simulink model "simulink_robo_fixo"  (R2014a)
settings: Solver=ode45  StartTime=0.0  StopTime=Tsim  RelTol=1e-3
values from neighbouring files (symbols this model uses):
  a = 0.0    (= 0)    [simula_robo_fixo.m]
  b = 0.2    [simula_robo_fixo.m]
  Ic = 1    [simula_robo_fixo.m]
  Kp = u(1)    [sfunc_adaptativo_J.m]    (also in simula_robo_fixo.m = 0.05)
  m = 10    [simula_robo_fixo.m]
  r = 0.07    [simula_robo_fixo.m]
  thetao = 0.0    (= 0)    [simula_robo_fixo.m]
  Ts = 0.1    [simula_robo_fixo.m]
  xo = -1.5    [simula_robo_fixo.m]
  yo = -2.5    [simula_robo_fixo.m]
libraries: vrlib x1
settings Model: PauseTimes=9  Creator=Fabricio  LastModifiedBy=Thiago Lobo
settings DataIOCC: SignalLoggingSaveFormat=ModelDataLogs
settings DebuggingCC: UnderspecifiedInitializationDetection=Classic  MultiTaskDSMMsg=warning  MultiTaskCondExecSysMsg=none  StateNameClashWarn=warning
settings RTWCC: IncludeERTFirstTime=on

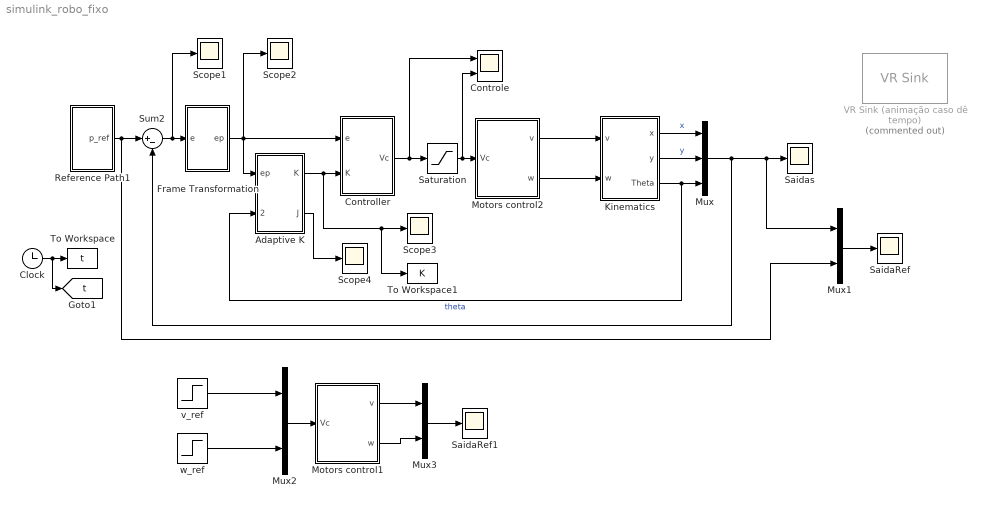
== system simulink_robo_fixo ==
  Adaptive K : Subsystem
  Clock : Clock
  Controle : Scope  NumInputPorts=2
      settings: ShowLegends=on  TimeRange=10  YMin=-5~-1e-08  YMax=20~1.3e-08  SaveName=ScopeData11
  Controller : Subsystem
  Frame Transformation : Subsystem
  Kinematics : Subsystem
  Motors control1 : Subsystem
  Motors control2 : Subsystem
  Mux : Mux  Inputs=3
  Mux1 : Mux  Inputs=2
  Mux2 : Mux  Inputs=2
  Mux3 : Mux  Inputs=2
  Reference Path1 : Subsystem
  SaidaRef : Scope
      settings: ShowLegends=on  TimeRange=10  YMin=-7.5  YMax=27.5  SaveName=ScopeData16
  SaidaRef1 : Scope
      settings: ShowLegends=on  TimeRange=10  YMin=-7.5  YMax=27.5  SaveName=ScopeData6
  Saidas : Scope
      settings: ShowLegends=on  TimeRange=10  YMax=100
  Saturation : Saturate  UpperLimit=[inf inf]  LowerLimit=-[inf inf]
  Scope{1..4} (4 alike) : Scope
      Scope1 settings: ShowLegends=on  TimeRange=10  SaveName=ScopeData2
      Scope2 settings: ShowLegends=on  TimeRange=10  SaveName=ScopeData9
      Scope3 settings: ShowLegends=on  TimeRange=10  YMax=300  SaveName=ScopeData4
      Scope4 settings: ShowLegends=on  TimeRange=10  SaveName=ScopeData8
  Sum2 : Sum  Inputs=|+-  SampleTime=Ts
  To Workspace : ToWorkspace  VariableName=t  SampleTime=Ts
  To Workspace1 : ToWorkspace  VariableName=K  SampleTime=Ts
  VR Sink (animação caso dê tempo) : vrlib/VR Sink  Commented=on  InstantiateOnLoad=on  SampleTime=0.1  ViewEnable=on  RemoteChange=off  RemoteView=on  AutoView=off  VideoDimensions=[]  AllowVariableSize=off
  v_ref : Step  Time=10  SampleTime=Ts
  w_ref : Step  Time=20  After=pi/2  SampleTime=Ts
  tag scope: t=global
  wires:
  Kinematics/2(y) -> Mux/2  "y"
  Kinematics/3(Theta) -> Adaptive K/2(Theta), Mux/3  "theta"
  Controller/1(Vc) -> Controle/1, Saturation/1
  Clock/1 -> To Workspace/1, [t]
  Mux/1 -> Mux1/1, Saidas/1, Sum2/2
  Sum2/1 -> Frame Transformation/1(e), Scope1/1
  Kinematics/1(x) -> Mux/1  "x"
  Motors control2/2(w) -> Kinematics/2(w)
  Motors control2/1(v) -> Kinematics/1(v)
  Frame Transformation/1(ep) -> Scope2/1, Adaptive K/1(ep), Controller/1(e)
  Adaptive K/2(J) -> Scope4/1
  Saturation/1 -> Motors control2/1(Vc), Controle/2
  Reference Path1/1(p_ref) -> Mux1/2, Sum2/1
  Mux1/1 -> SaidaRef/1
  Mux2/1 -> Motors control1/1(Vc)
  v_ref/1 -> Mux2/1
  w_ref/1 -> Mux2/2
  Mux3/1 -> SaidaRef1/1
  Motors control1/1(v) -> Mux3/1
  Motors control1/2(w) -> Mux3/2
  Adaptive K/1(K) -> To Workspace1/1, Scope3/1, Controller/2(K)

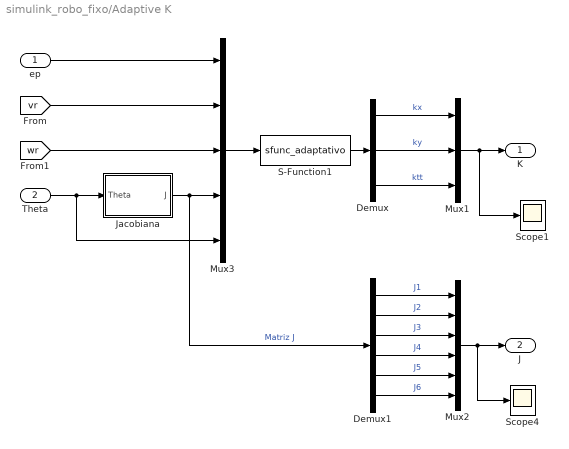
== system simulink_robo_fixo/Adaptive K ==
  ep : Inport
  Theta : Inport  Port=2
  Demux : Demux  Outputs=3
  Demux1 : Demux  Outputs=6
  Jacobiana : Subsystem
  Mux1 : Mux  Inputs=3
  Mux2 : Mux  Inputs=6
  Mux3 : Mux  Inputs=5
  S-Function1 : S-Function  FunctionName=sfunc_adaptativo  Parameters=Ts  EnableBusSupport=off
  Scope1 : Scope
      settings: ShowLegends=on  TimeRange=10  YMin=-100  YMax=220  SaveName=ScopeData14
  Scope4 : Scope
      settings: ShowLegends=on  TimeRange=10  SaveName=ScopeData13
  K : Outport
  J : Outport  Port=2
  wires:
  Mux3/1 -> S-Function1/1
  [vr] -> Mux3/2
  [wr] -> Mux3/3
  S-Function1/1 -> Demux/1
  Demux/3 -> Mux1/3  "ktt"
  Demux/2 -> Mux1/2  "ky"
  Demux/1 -> Mux1/1  "kx"
  ep/1 -> Mux3/1
  Theta/1 -> Mux3/5, Jacobiana/1(Theta)
  Jacobiana/1(J) -> Demux1/1, Mux3/4  "Matriz J"
  Demux1/3 -> Mux2/3  "J3"
  Demux1/2 -> Mux2/2  "J2"
  Demux1/1 -> Mux2/1  "J1"
  Demux1/4 -> Mux2/4  "J4"
  Demux1/5 -> Mux2/5  "J5"
  Demux1/6 -> Mux2/6  "J6"
  Mux1/1 -> Scope1/1, K/1
  Mux2/1 -> Scope4/1, J/1

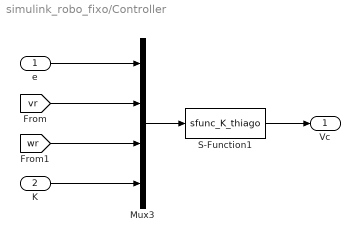
== system simulink_robo_fixo/Controller ==
  e : Inport
  K : Inport  Port=2
  Mux3 : Mux
  S-Function1 : S-Function  FunctionName=sfunc_K_thiago  Parameters=Ts  EnableBusSupport=off
  Vc : Outport
  wires:
  Mux3/1 -> S-Function1/1
  [vr] -> Mux3/2
  [wr] -> Mux3/3
  S-Function1/1 -> Vc/1
  e/1 -> Mux3/1
  K/1 -> Mux3/4

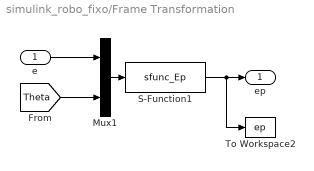
== system simulink_robo_fixo/Frame Transformation ==
  e : Inport
  Mux1 : Mux  Inputs=2
  S-Function1 : S-Function  FunctionName=sfunc_Ep  Parameters=Ts  EnableBusSupport=off
  To Workspace2 : ToWorkspace  VariableName=ep  SampleTime=Ts
  ep : Outport
  wires:
  S-Function1/1 -> To Workspace2/1, ep/1
  Mux1/1 -> S-Function1/1
  e/1 -> Mux1/1
  [Theta] -> Mux1/2

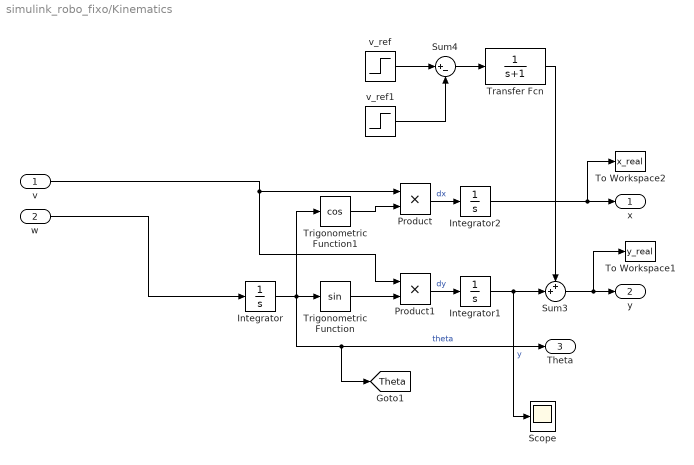
== system simulink_robo_fixo/Kinematics ==
  v : Inport
  w : Inport  Port=2
  Integrator : Integrator  InitialCondition=thetao
  Integrator1 : Integrator  InitialCondition=yo
  Integrator2 : Integrator  InitialCondition=xo
  Product : Product
  Product1 : Product
  Scope : Scope
      settings: TimeRange=10
  Sum3 : Sum  Inputs=++|
  Sum4 : Sum  Inputs=|+-
  To Workspace1 : ToWorkspace  VariableName=y_real  SampleTime=Ts
  To Workspace2 : ToWorkspace  VariableName=x_real  SampleTime=Ts
  Transfer Fcn : TransferFcn  Denominator=[1 1]
  Trigonometric Function : Trigonometry
  Trigonometric Function1 : Trigonometry  Operator=cos
  v_ref : Step  Time=80000  After=-0.1  SampleTime=Ts
  v_ref1 : Step  Time=810000  After=-0.1  SampleTime=Ts
  x : Outport
  y : Outport  Port=2
  Theta : Outport  Port=3
  tag scope: Theta=global
  wires:
  Trigonometric Function1/1 -> Product/2
  Product/1 -> Integrator2/1  "dx"
  Integrator/1 -> [Theta], Theta/1, Trigonometric Function1/1, Trigonometric Function/1  "theta"
  Integrator1/1 -> Sum3/2, Scope/1  "y"
  Product1/1 -> Integrator1/1  "dy"
  Trigonometric Function/1 -> Product1/2
  v_ref/1 -> Sum4/1
  v_ref1/1 -> Sum4/2
  Sum4/1 -> Transfer Fcn/1
  Integrator2/1 -> To Workspace2/1, x/1
  Sum3/1 -> To Workspace1/1, y/1
  Transfer Fcn/1 -> Sum3/1
  w/1 -> Integrator/1
  v/1 -> Product1/1, Product/1

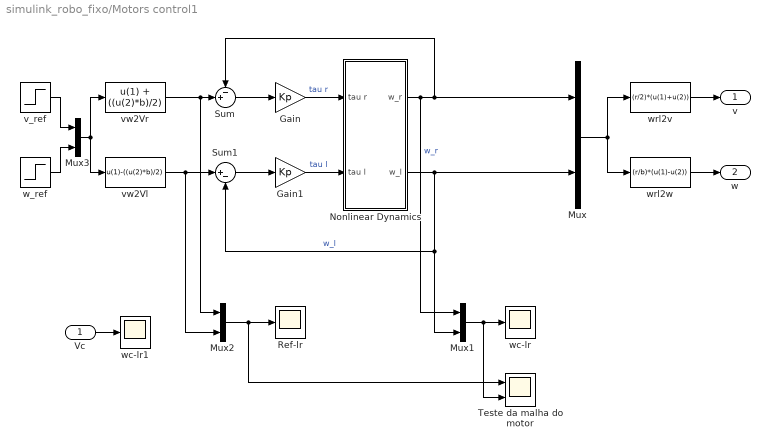
== system simulink_robo_fixo/Motors control1 ==
  Vc : Inport
  Gain : Gain  Gain=Kp
  Gain1 : Gain  Gain=Kp
  Mux{,1..3} (4 alike) : Mux  Inputs=2
  Nonlinear Dynamics : Subsystem
  Ref-lr : Scope
      settings: YMax=20  SaveName=ScopeData7
  Sum : Sum  Inputs=-+|
  Sum1 : Sum  Inputs=|+-
  Teste da malha do motor : Scope  NumInputPorts=2
      settings: YMin=-5~-5  YMax=5~5  SaveName=ScopeData10
  v_ref : Step  Time=10  SampleTime=Ts
  vw2Vl : Fcn  Expr=u(1)-((u(2)*b)/2)
  vw2Vr : Fcn  Expr=u(1) + ((u(2)*b)/2)
  w_ref : Step  Time=12  After=pi/2  SampleTime=Ts
  wc-lr : Scope
      settings: YMax=20  SaveName=ScopeData5
  wc-lr1 : Scope
      settings: YMax=20  SaveName=ScopeData3
  wrl2v : Fcn  Expr=(r/2)*(u(1)+u(2))
  wrl2w : Fcn  Expr=(r/b)*(u(1)-u(2))
  v : Outport
  w : Outport  Port=2
  wires:
  Gain/1 -> Nonlinear Dynamics/1(tau r)  "tau r"
  Sum/1 -> Gain/1
  Gain1/1 -> Nonlinear Dynamics/2(tau l)  "tau l"
  Sum1/1 -> Gain1/1
  Nonlinear Dynamics/1(w_r) -> Mux/1, Sum/1, Mux1/1  "w_r"
  Nonlinear Dynamics/2(w_l) -> Mux1/2, Sum1/2, Mux/2  "w_l"
  vw2Vr/1 -> Mux2/1, Sum/2
  vw2Vl/1 -> Sum1/1, Mux2/2
  Mux1/1 -> Teste da malha do motor/2, wc-lr/1
  Mux2/1 -> Teste da malha do motor/1, Ref-lr/1
  Mux/1 -> wrl2w/1, wrl2v/1
  wrl2v/1 -> v/1
  wrl2w/1 -> w/1
  w_ref/1 -> Mux3/2
  v_ref/1 -> Mux3/1
  Mux3/1 -> vw2Vl/1, vw2Vr/1
  Vc/1 -> wc-lr1/1

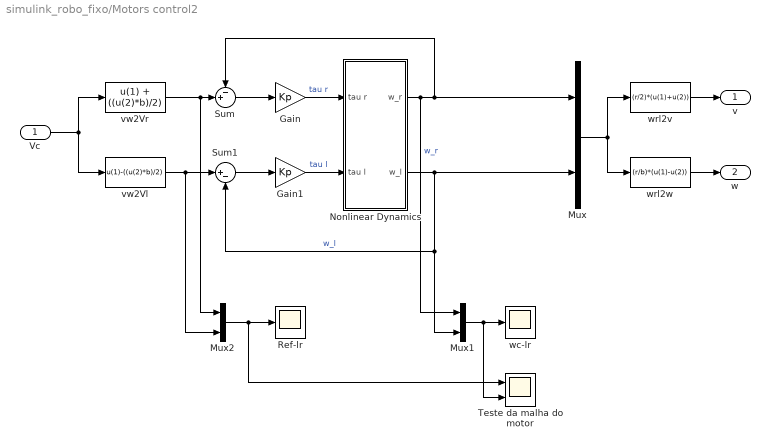
== system simulink_robo_fixo/Motors control2 ==
  Vc : Inport
  Gain : Gain  Gain=Kp
  Gain1 : Gain  Gain=Kp
  Mux : Mux  Inputs=2
  Mux1 : Mux  Inputs=2
  Mux2 : Mux  Inputs=2
  Nonlinear Dynamics : Subsystem
  Ref-lr : Scope
      settings: YMax=20  SaveName=ScopeData7
  Sum : Sum  Inputs=-+|
  Sum1 : Sum  Inputs=|+-
  Teste da malha do motor : Scope  NumInputPorts=2
      settings: YMin=-5~-5  YMax=5~5  SaveName=ScopeData10
  vw2Vl : Fcn  Expr=u(1)-((u(2)*b)/2)
  vw2Vr : Fcn  Expr=u(1) + ((u(2)*b)/2)
  wc-lr : Scope
      settings: YMax=20  SaveName=ScopeData5
  wrl2v : Fcn  Expr=(r/2)*(u(1)+u(2))
  wrl2w : Fcn  Expr=(r/b)*(u(1)-u(2))
  v : Outport
  w : Outport  Port=2
  wires:
  Gain/1 -> Nonlinear Dynamics/1(tau r)  "tau r"
  Sum/1 -> Gain/1
  Gain1/1 -> Nonlinear Dynamics/2(tau l)  "tau l"
  Sum1/1 -> Gain1/1
  Nonlinear Dynamics/1(w_r) -> Mux/1, Sum/1, Mux1/1  "w_r"
  Nonlinear Dynamics/2(w_l) -> Mux1/2, Sum1/2, Mux/2  "w_l"
  vw2Vr/1 -> Mux2/1, Sum/2
  vw2Vl/1 -> Sum1/1, Mux2/2
  Mux1/1 -> Teste da malha do motor/2, wc-lr/1
  Mux2/1 -> Teste da malha do motor/1, Ref-lr/1
  Mux/1 -> wrl2w/1, wrl2v/1
  wrl2v/1 -> v/1
  wrl2w/1 -> w/1
  Vc/1 -> vw2Vr/1, vw2Vl/1

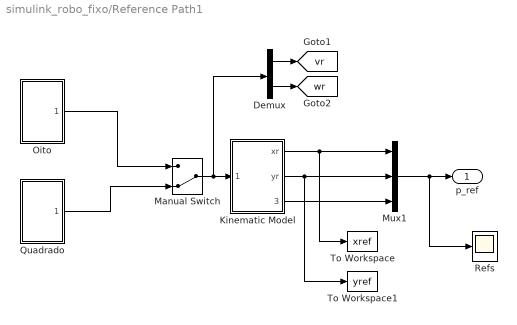
== system simulink_robo_fixo/Reference Path1 ==
  Demux : Demux  Outputs=2
  Kinematic Model : Subsystem
  Manual Switch : ManualSwitch  CurrentSetting=0
  Mux1 : Mux  Inputs=3
  Oito : Subsystem
  Quadrado : Subsystem
  Refs : Scope
      settings: ShowLegends=on  TimeRange=10  SaveName=ScopeData12
  To Workspace : ToWorkspace  VariableName=xref  SampleTime=Ts
  To Workspace1 : ToWorkspace  VariableName=yref  SampleTime=Ts
  p_ref : Outport
  tag scope: vr=global, wr=global
  wires:
  Kinematic Model/1(xr) -> To Workspace/1, Mux1/1
  Kinematic Model/3(thetar) -> Mux1/3
  Mux1/1 -> Refs/1, p_ref/1
  Kinematic Model/2(yr) -> To Workspace1/1, Mux1/2
  Oito/1(vw_ref) -> Manual Switch/1
  Quadrado/1(vw_ref) -> Manual Switch/2
  Demux/1 -> [vr]
  Demux/2 -> [wr]
  Manual Switch/1 -> Demux/1, Kinematic Model/1(vw_ref)

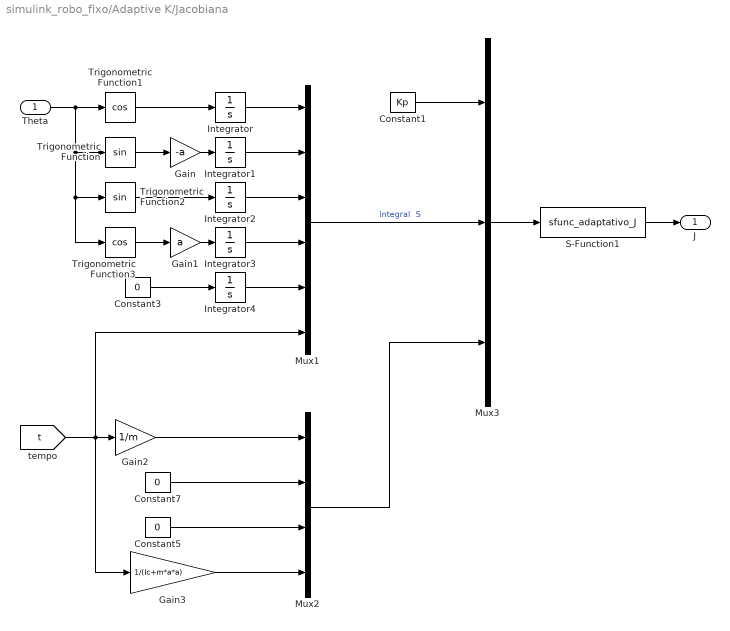
== system simulink_robo_fixo/Adaptive K/Jacobiana ==
  Theta : Inport
  Constant1 : Constant  Value=Kp  SampleTime=Ts
  Constant3 : Constant  Value=0  SampleTime=Ts
  Constant5 : Constant  Value=0  SampleTime=Ts
  Constant7 : Constant  Value=0  SampleTime=Ts
  Gain : Gain  Gain=-a
  Gain1 : Gain  Gain=a
  Gain2 : Gain  Gain=1/m
  Gain3 : Gain  Gain=1/(Ic+m*a*a)
  Integrator{,1..4} (5 alike) : Integrator
  Mux1 : Mux  Inputs=6
  Mux2 : Mux
  Mux3 : Mux  Inputs=3
  S-Function1 : S-Function  FunctionName=sfunc_adaptativo_J  Parameters=Ts  EnableBusSupport=off
  Trigonometric Function : Trigonometry
  Trigonometric Function1 : Trigonometry  Operator=cos
  Trigonometric Function2 : Trigonometry
  Trigonometric Function3 : Trigonometry  Operator=cos
  J : Outport
  wires:
  Mux3/1 -> S-Function1/1
  S-Function1/1 -> J/1
  Constant3/1 -> Integrator4/1
  Trigonometric Function1/1 -> Integrator/1
  Integrator/1 -> Mux1/1
  Integrator2/1 -> Mux1/3
  Integrator3/1 -> Mux1/4
  Integrator4/1 -> Mux1/5
  Integrator1/1 -> Mux1/2
  Gain2/1 -> Mux2/1
  Constant5/1 -> Mux2/3
  Gain3/1 -> Mux2/4
  Constant7/1 -> Mux2/2
  [t] -> Gain2/1, Mux1/6, Gain3/1
  Trigonometric Function/1 -> Gain/1
  Gain/1 -> Integrator1/1
  Theta/1 -> Trigonometric Function1/1, Trigonometric Function/1, Trigonometric Function2/1, Trigonometric Function3/1
  Trigonometric Function2/1 -> Integrator2/1
  Trigonometric Function3/1 -> Gain1/1
  Gain1/1 -> Integrator3/1
  Constant1/1 -> Mux3/1
  Mux1/1 -> Mux3/2  "integral  S"
  Mux2/1 -> Mux3/3

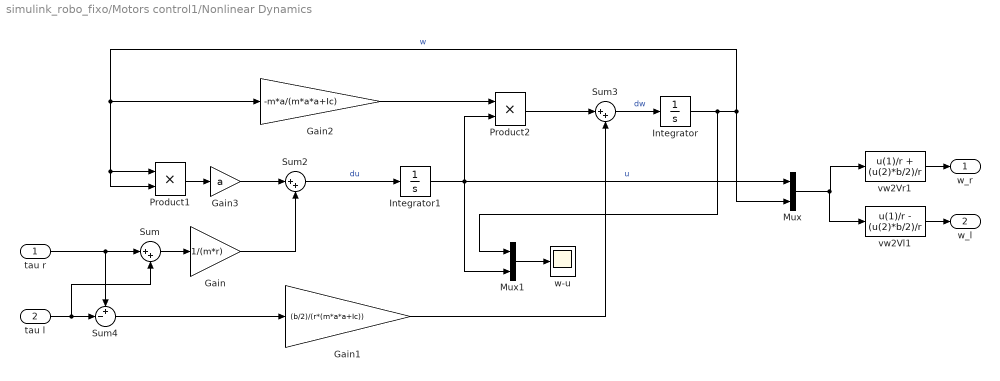
== system simulink_robo_fixo/Motors control1/Nonlinear Dynamics ==
  tau r : Inport
  tau l : Inport  Port=2
  Gain : Gain  Gain=1/(m*r)
  Gain1 : Gain  Gain=(b/2)/(r*(m*a*a+Ic))
  Gain2 : Gain  Gain=-m*a/(m*a*a+Ic)
  Gain3 : Gain  Gain=a
  Integrator : Integrator
  Integrator1 : Integrator
  Mux : Mux  Inputs=2
  Mux1 : Mux  Inputs=2
  Product1 : Product
  Product2 : Product  SampleTime=Ts
  Sum : Sum  Inputs=|++
  Sum2 : Sum  Inputs=|++
  Sum3 : Sum  Inputs=|++
  Sum4 : Sum  Inputs=+-|
  vw2Vl1 : Fcn  Expr=u(1)/r - (u(2)*b/2)/r
  vw2Vr1 : Fcn  Expr=u(1)/r + (u(2)*b/2)/r
  w-u : Scope
      settings: TimeRange=10  SaveName=ScopeData15
  w_r : Outport
  w_l : Outport  Port=2
  wires:
  tau r/1 -> Sum4/1, Sum/1
  Sum/1 -> Gain/1
  Product1/1 -> Gain3/1
  Gain3/1 -> Sum2/1
  Gain/1 -> Sum2/2
  Product2/1 -> Sum3/1
  Gain1/1 -> Sum3/2
  Integrator1/1 -> Mux1/2, Mux/1, Product2/2  "u"
  Sum2/1 -> Integrator1/1  "du"
  Sum3/1 -> Integrator/1  "dw"
  Integrator/1 -> Mux1/1, Mux/2, Gain2/1, Product1/1, Product1/2  "w"
  Gain2/1 -> Product2/1
  Sum4/1 -> Gain1/1
  tau l/1 -> Sum/2, Sum4/2
  vw2Vr1/1 -> w_r/1
  vw2Vl1/1 -> w_l/1
  Mux/1 -> vw2Vl1/1, vw2Vr1/1
  Mux1/1 -> w-u/1

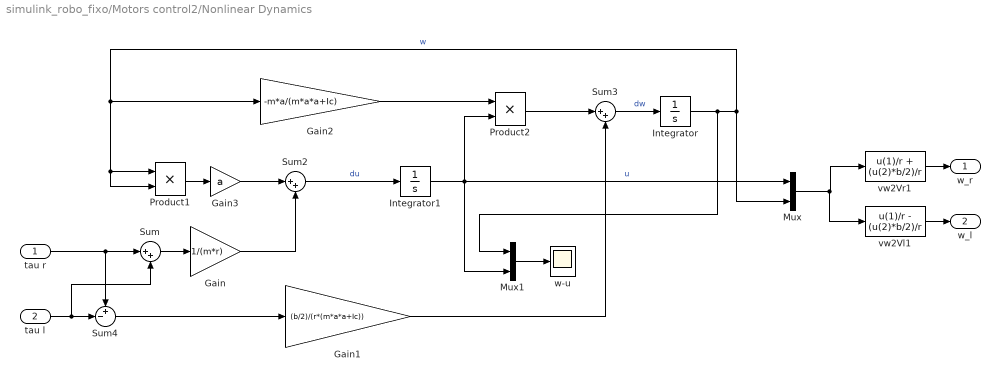
== system simulink_robo_fixo/Motors control2/Nonlinear Dynamics ==
  tau r : Inport
  tau l : Inport  Port=2
  Gain : Gain  Gain=1/(m*r)
  Gain1 : Gain  Gain=(b/2)/(r*(m*a*a+Ic))
  Gain2 : Gain  Gain=-m*a/(m*a*a+Ic)
  Gain3 : Gain  Gain=a
  Integrator : Integrator
  Integrator1 : Integrator
  Mux : Mux  Inputs=2
  Mux1 : Mux  Inputs=2
  Product1 : Product
  Product2 : Product  SampleTime=Ts
  Sum : Sum  Inputs=|++
  Sum2 : Sum  Inputs=|++
  Sum3 : Sum  Inputs=|++
  Sum4 : Sum  Inputs=+-|
  vw2Vl1 : Fcn  Expr=u(1)/r - (u(2)*b/2)/r
  vw2Vr1 : Fcn  Expr=u(1)/r + (u(2)*b/2)/r
  w-u : Scope
      settings: TimeRange=10  SaveName=ScopeData15
  w_r : Outport
  w_l : Outport  Port=2
  wires:
  tau r/1 -> Sum4/1, Sum/1
  Sum/1 -> Gain/1
  Product1/1 -> Gain3/1
  Gain3/1 -> Sum2/1
  Gain/1 -> Sum2/2
  Product2/1 -> Sum3/1
  Gain1/1 -> Sum3/2
  Integrator1/1 -> Mux1/2, Mux/1, Product2/2  "u"
  Sum2/1 -> Integrator1/1  "du"
  Sum3/1 -> Integrator/1  "dw"
  Integrator/1 -> Mux1/1, Mux/2, Gain2/1, Product1/1, Product1/2  "w"
  Gain2/1 -> Product2/1
  Sum4/1 -> Gain1/1
  tau l/1 -> Sum/2, Sum4/2
  vw2Vr1/1 -> w_r/1
  vw2Vl1/1 -> w_l/1
  Mux/1 -> vw2Vl1/1, vw2Vr1/1
  Mux1/1 -> w-u/1

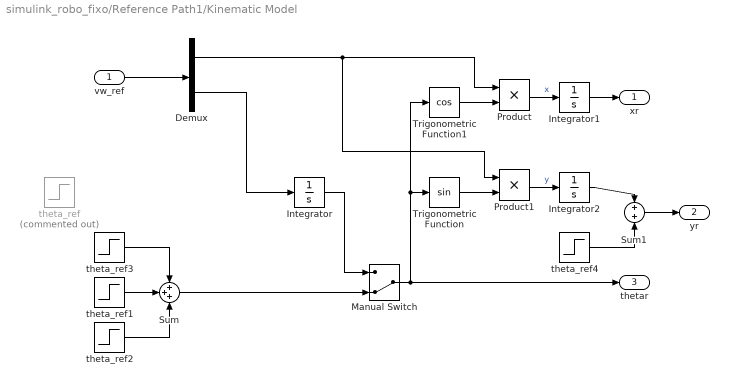
== system simulink_robo_fixo/Reference Path1/Kinematic Model ==
  vw_ref : Inport
  Demux : Demux  Outputs=2
  Integrator : Integrator
  Integrator1 : Integrator
  Integrator2 : Integrator
  Manual Switch : ManualSwitch  CurrentSetting=0
  Product : Product
  Product1 : Product
  Sum : Sum  Inputs=+++
  Sum1 : Sum
  Trigonometric Function : Trigonometry
  Trigonometric Function1 : Trigonometry  Operator=cos
  theta_ref : Step  Commented=on  Time=200  Before=pi/2  After=pi
  theta_ref1 : Step  Time=20  After=pi/2  SampleTime=Ts
  theta_ref2 : Step  Time=30  After=pi/2  SampleTime=Ts
  theta_ref3 : Step  Time=10  After=pi/2  SampleTime=Ts
  theta_ref4 : Step  Time=10000  SampleTime=Ts
  xr : Outport
  yr : Outport  Port=2
  thetar : Outport  Port=3
  wires:
  Trigonometric Function1/1 -> Product/2
  Product/1 -> Integrator1/1  "x"
  Integrator/1 -> Manual Switch/1
  Product1/1 -> Integrator2/1  "y"
  Trigonometric Function/1 -> Product1/2
  Demux/1 -> Product/1, Product1/1
  Demux/2 -> Integrator/1
  vw_ref/1 -> Demux/1
  theta_ref1/1 -> Sum/2
  theta_ref2/1 -> Sum/3
  Sum/1 -> Manual Switch/2
  Manual Switch/1 -> Trigonometric Function1/1, Trigonometric Function/1, thetar/1
  theta_ref3/1 -> Sum/1
  Integrator1/1 -> xr/1
  Integrator2/1 -> Sum1/1
  Sum1/1 -> yr/1
  theta_ref4/1 -> Sum1/2

== system simulink_robo_fixo/Reference Path1/Oito ==
  Mux : Mux  Inputs=2
  v_ref : Step  Before=1  SampleTime=Ts
  w_ref : Step  Time=63  Before=0.1  After=-0.1  SampleTime=Ts
  vw_ref : Outport
  wires:
  v_ref/1 -> Mux/1
  w_ref/1 -> Mux/2
  Mux/1 -> vw_ref/1

== system simulink_robo_fixo/Reference Path1/Quadrado ==
  Mux : Mux  Inputs=2
  vref : Constant  SampleTime=Ts
  wref : Constant  Value=0  SampleTime=Ts
  vw_ref : Outport
  wires:
  vref/1 -> Mux/1
  wref/1 -> Mux/2
  Mux/1 -> vw_ref/1
